simulink model "ComparaModelos"  (R2023b)
settings: Solver=VariableStepAuto  StartTime=0.0  StopTime=10.0  RelTol=1e-3
settings Model: Creator=marqu  LastModifiedBy=marqu

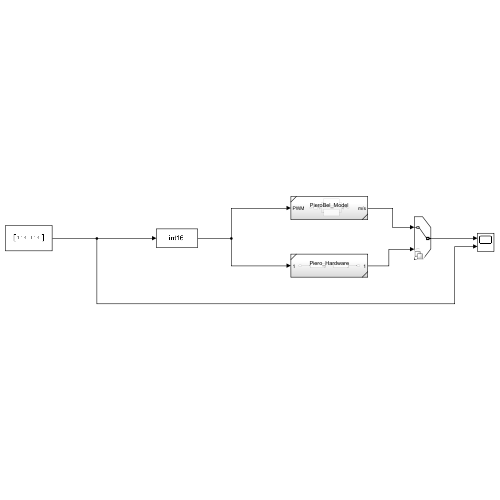
[thumbnail: Simulink's stored preview of the top-level diagram]
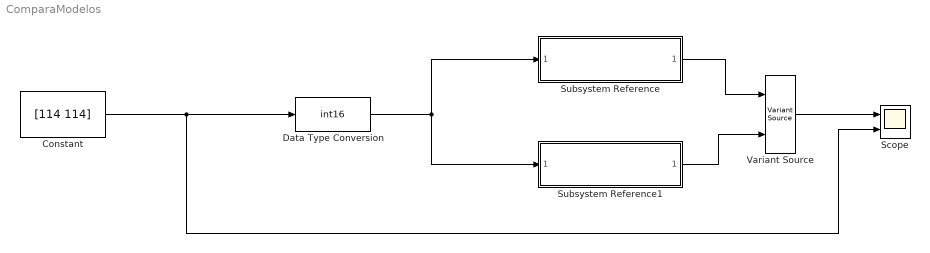
== system ComparaModelos ==
  Constant : Constant  Value=[114 114]  VectorParams1D=off
  Data Type Conversion : DataTypeConversion  OutDataTypeStr=int16  SaturateOnIntegerOverflow=off  RndMeth=Floor
  Scope : Scope  NumInputPorts=2
  Subsystem Reference : Subsystem  ReferencedSubsystem=PieroBel_Model
  Subsystem Reference1 : Subsystem  ReferencedSubsystem=Piero_Hardware
  Variant Source : VariantSource
  wires:
  Variant Source/1 -> Scope/1
  Data Type Conversion/1 -> Subsystem Reference/1, Subsystem Reference1/1
  Subsystem Reference1/1 -> Variant Source/2
  Subsystem Reference/1 -> Variant Source/1
  Constant/1 -> Data Type Conversion/1, Scope/2
